simulink model "ejercicio_3"  (R2020b)
settings: Solver=ode4  StartTime=0.0  StopTime=30.0  FixedStep=0.05  MaxStep=0.01  RelTol=1e-3
settings Model: EnablePacing=on  Creator=alexa  LastModifiedBy=alexa

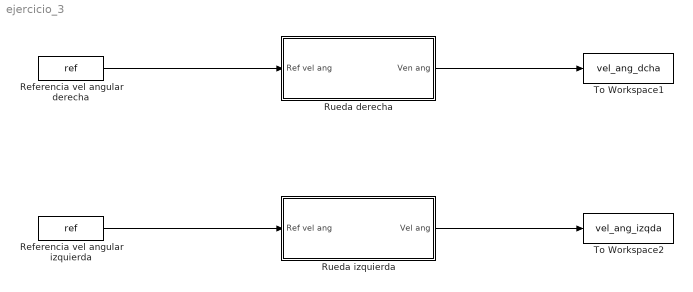
== system ejercicio_3 ==
  Referencia vel angular derecha : FromWorkspace  VariableName=ref
  Referencia vel angular izquierda : FromWorkspace  VariableName=ref
  Rueda derecha : Subsystem
  Rueda izquierda : Subsystem
  To Workspace1 : ToWorkspace  VariableName=vel_ang_dcha  SaveFormat=Timeseries  SampleTime=-1
  To Workspace2 : ToWorkspace  VariableName=vel_ang_izqda  SaveFormat=Timeseries  SampleTime=-1
  wires:
  Referencia vel angular derecha/1 -> Rueda derecha/1(Ref vel ang)
  Rueda derecha/1(Ven ang) -> To Workspace1/1
  Rueda izquierda/1(Vel ang) -> To Workspace2/1
  Referencia vel angular izquierda/1 -> Rueda izquierda/1(Ref vel ang)

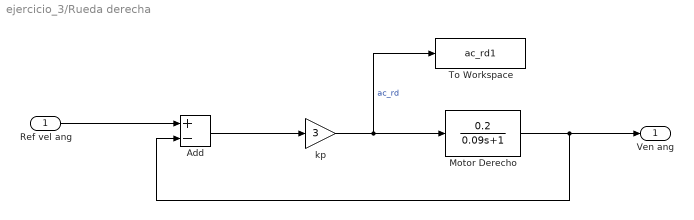
== system ejercicio_3/Rueda derecha ==
  Ref vel ang : Inport
  Add : Sum  Inputs=+-
  Motor Derecho : TransferFcn  Numerator=[0.2]  Denominator=[0.09 1]
  To Workspace : ToWorkspace  VariableName=ac_rd1  SaveFormat=Timeseries  SampleTime=-1
  kp : Gain  Gain=3
  Ven ang : Outport
  wires:
  Add/1 -> kp/1
  kp/1 -> To Workspace/1, Motor Derecho/1  "ac_rd"
  Motor Derecho/1 -> Ven ang/1, Add/2
  Ref vel ang/1 -> Add/1

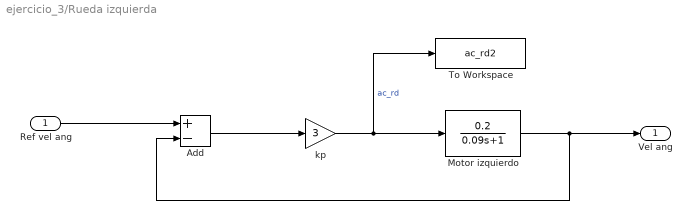
== system ejercicio_3/Rueda izquierda ==
  Ref vel ang : Inport
  Add : Sum  Inputs=+-
  Motor izquierdo : TransferFcn  Numerator=[0.2]  Denominator=[0.09 1]
  To Workspace : ToWorkspace  VariableName=ac_rd2  SaveFormat=Timeseries  SampleTime=-1
  kp : Gain  Gain=3
  Vel ang : Outport
  wires:
  Add/1 -> kp/1
  kp/1 -> To Workspace/1, Motor izquierdo/1  "ac_rd"
  Motor izquierdo/1 -> Vel ang/1, Add/2
  Ref vel ang/1 -> Add/1
